simulink model "Ae483_project"  (R2018a)
settings: Solver=ode15s  StartTime=0.0  StopTime=50  RelTol=1e-4
values from neighbouring files (symbols this model uses):
  A_10_ang = [-1.3336 -0.5124 0.1399 ... (first row only)    [Ae483Project.m]
  A_10_ang_ob = bsxfun(@times, A_10_ang, [1.02; 1.04; 1.06])    [Ae483Project.m]
  A_10_full = [-0.006289	0.032720	1.318244	-32.063538	0.001827	-0.977238	0.000000	0.000733 ... (first row only)    [Ae483Project.m]
  A_80_ang = [-1.4979 -0.2372 0.4009 ... (first row only)    [Ae483Project.m]
  A_80_ang_ob = bsxfun(@times, A_80_ang, [1.02; 1.04; 1.06])    [Ae483Project.m]
  A_80_full = [-0.107611	0.120068	11.216902	-32.054340	0.007203	-0.521417	0.000000	-0.035677 ... (first row only)    [Ae483Project.m]
  B_10_ang = [-0.1712 16.8793 3.8113 ... (first row only)    [Ae483Project.m]
  B_10_ang_ob = bsxfun(@times, B_10_ang, [1.02; 1.04; 1.06])    [Ae483Project.m]
  B_10_full = [32.104822	29.961036	0.359934	0.000000 ... (first row only)    [Ae483Project.m]
  B_80_ang = [3.4190 17.0171 5.3246 ... (first row only)    [Ae483Project.m]
  B_80_ang_ob = bsxfun(@times, B_80_ang, [1.02; 1.04; 1.06])    [Ae483Project.m]
  B_80_full = [17.121858	64.081477	0.195110	0.000000 ... (first row only)    [Ae483Project.m]
  K_10 = B_10_ang^-1*(A_10_ang-A_d_ang)*C_ang^-1    [Ae483Project.m]
  K_80 = B_80_ang^-1*(A_80_ang-A_d_ang)*C_ang^-1    [Ae483Project.m]
  Ke_ang_10 = double(sym([ke1_ang_10; ke2_ang_10; ke3_ang_10]))    [Ae483Project.m]
  Ke_ang_80 = double(sym([ke1_ang_80; ke2_ang_80; ke3_ang_80]))    [Ae483Project.m]
  L_bv_10 = [cos(theta_10)*cos(psi_10), cos(theta_10)*sin(psi_10), -sin(theta_10) ... (first row only)    [Ae483Project.m]
  L_vb_10 = L_bv_10'    [Ae483Project.m]
undefined symbols (not defined in the file or in its folder): K_lqr_10, K_lqr_10_full, K_lqr_80, K_lqr_80_full
(part 1 of 2)
settings Model: Creator=90554  LastModifiedBy=90554

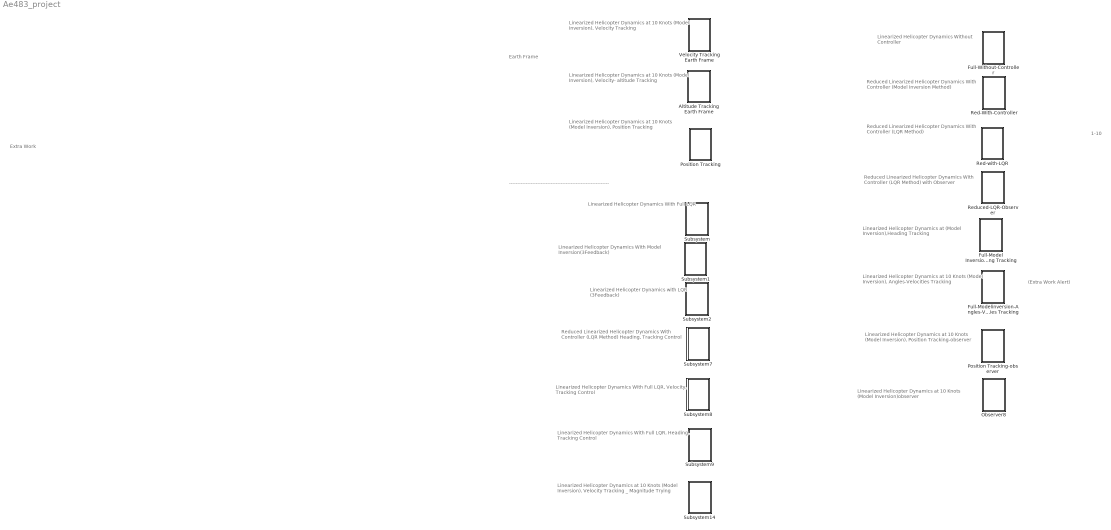
== system Ae483_project ==
  note: ------------------------------------------------------------
  note: (Extra Work Alert)
  note: 1-10
  note: Linearized Helicopter
      | Dynamics
      | Without Controller
  note: Reduced Linearized Helicopter
      | Dynamics
      | With Controller
      | (Model Inversion Method)
  note: Reduced Linearized Helicopter
      | Dynamics
      | With Controller
      | (LQR Method)
  note: Reduced Linearized Helicopter
      | Dynamics
      | With Controller
      | (LQR Method) with Observer
  note: Linearized Helicopter
      | Dynamics at
      | (Model Inversion),Heading Tracking
  note: Linearized Helicopter
      | Dynamics at 10 Knots
      | (Model Inversion), Angles-Velocities Tracking
  note: Linearized Helicopter
      | Dynamics at 10 Knots
      | (Model Inversion), Velocity Tracking
  note: Earth Frame
  note: Linearized Helicopter
      | Dynamics at 10 Knots
      | (Model Inversion), Velocity- altitude Tracking
  note: Reduced Linearized Helicopter
      | Dynamics
      | With Controller
      | (LQR Method) Heading, Tracking Control
  note: Linearized Helicopter
      | Dynamics
      | With Full LQR, Heading, Tracking Control
  note: Linearized Helicopter
      | Dynamics
      | With Full LQR, Velocity, Tracking Control
  note: Linearized Helicopter
      | Dynamics with
      | LQR (3Feedback)
  note: Linearized Helicopter
      | Dynamics
      | With Model Inversion(3Feedback)
  note: Linearized Helicopter
      | Dynamics
      | With Full LQR
  note: Linearized Helicopter
      | Dynamics at 10 Knots
      | (Model Inversion), Velocity Tracking _ Magnitude Trying
  note: Extra Work
  note: Linearized Helicopter
      | Dynamics at 10 Knots
      | (Model Inversion), Position Tracking
  note: Linearized Helicopter
      | Dynamics at 10 Knots
      | (Model Inversion), Position Tracking-observer
  note: Linearized Helicopter
      | Dynamics at 10 Knots
      | (Model Inversion)observer
  Altitude Tracking Earth Frame : Subsystem
  Full-Model Inversion-Heading Tracking : Subsystem
  Full-Modelinversion-Angles-Velocities Tracking : Subsystem
  Full-Without-Controller : Subsystem
  Observer8 : Subsystem
  Position Tracking : Subsystem
  Position Tracking-observer : Subsystem
  Red-With-Controller : Subsystem
  Red-with-LQR : Subsystem
  Reduced-LQR-Observer : Subsystem
  Subsystem : Subsystem
  Subsystem1 : Subsystem
  Subsystem14 : Subsystem
  Subsystem2 : Subsystem
  Subsystem7 : Subsystem
  Subsystem8 : Subsystem
  Subsystem9 : Subsystem
  Velocity Tracking Earth Frame : Subsystem

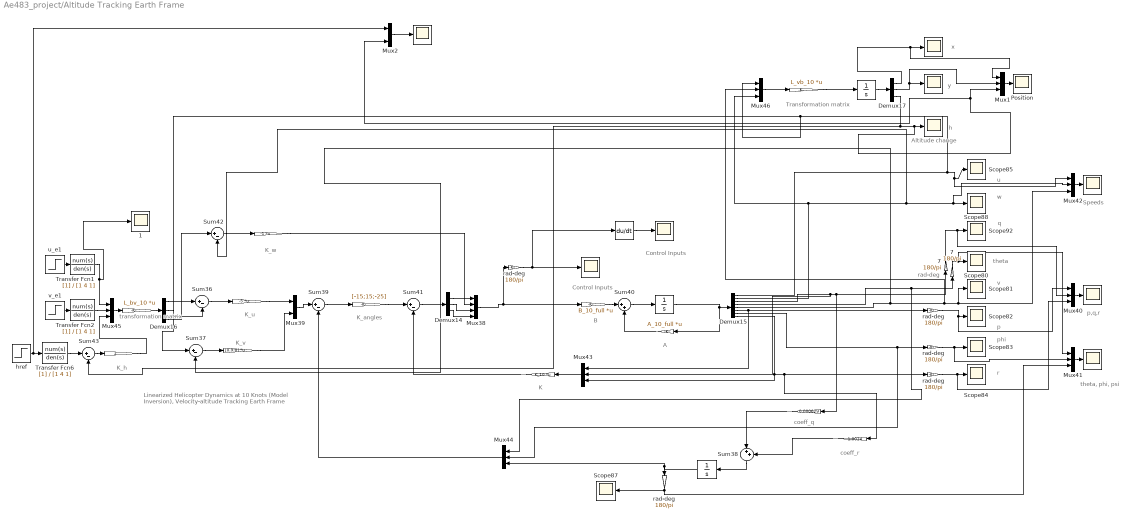
== system Ae483_project/Altitude Tracking Earth Frame ==
  note: x
  note: y
  note: h
  note: Transformation
      |       matrix
  note: Altitude change
  note: K_angles
  note: K_u
  note: K_w
  note: K_v
  note: transformation
      |      matrix
  note: K_h
  note: coeff_r
  note: coeff_q
  note: Control Inputs
  note: Control Inputs
  note: B
  note: K
  note: Linearized Helicopter
      | Dynamics at 10 Knots
      | (Model Inversion), Velocity-altitude Tracking Earth Frame
  note: w
  note: u
  note: p,q,r
  note: Speeds
  note: A
  note: phi
  note: theta
  note: p
  note: rad-deg
  note: theta, phi, psi
  note: r
  note: v
  note: q
  "    " : Gain  Gain=B_10_full  Multiplication=Matrix(K*u)
  "     " : Gain  Gain=2
  "       " : Gain  Gain=K_10  Multiplication=Matrix(K*u)
  "            " : Scope
  "             " : Integrator
  "              " : Scope
  "                " : Gain  Gain=1.0024
  "                    " : Gain  Gain=-1  Multiplication=Matrix(K*u)
  "                           " : Gain  Gain=A_10_full  Multiplication=Matrix(K*u)
  "                                    " : Gain  Gain=0.000629
  "                                      " : Gain  Gain=L_bv_10  Multiplication=Matrix(K*u)
  "                                              " : Integrator
  "                                               " : Derivative
  "                                                " : Scope
  "                                                          " : Scope
  "                                                                     " : Scope
  "                                                                        " : Integrator
  "                                                                         " : Gain  Gain=-5  Multiplication=Matrix(K*u)
  "                                                                                " : Gain  Gain=[-15;15;-25]
  "                                                                                 " : Scope
  "                                                                                   " : Scope
  "                                                                                     " : Scope
  "                                                                                       " : Scope
  "                                                                                        " : Gain  Gain=[0.9;0]  Multiplication=Matrix(K*u)
  "                                                                                                                                                      " : Gain  Gain=L_vb_10  Multiplication=Matrix(K*u)
  "                                                          1" : Scope
  "                                        Position                                            " : Scope
  "    7" : Gain  Gain=180/pi
  " 7" : Gain  Gain=180/pi
  " rad-deg   " : Gain  Gain=180/pi
  Demux14 : Demux  Outputs=3
  Demux15 : Demux  Outputs=8
  Demux16 : Demux  Outputs=3
  Demux17 : Demux  Outputs=3
  Mux{1,40..46} (8 alike) : Mux  Inputs=3
  Mux2 : Mux  Inputs=2
  Mux38 : Mux
  Mux39 : Mux  Inputs=2
  Scope{80..85,87..88,92} (9 alike) : Scope
  Sum{36..37,39,41..43} (6 alike) : Sum  Inputs=|+-
  Sum38 : Sum  Inputs=|++
  Sum40 : Sum  Inputs=|++
  Transfer Fcn1 : TransferFcn  Denominator=[1 4 1]
  Transfer Fcn2 : TransferFcn  Denominator=[1 4 1]
  Transfer Fcn6 : TransferFcn  Denominator=[1 4 1]
  href : Step  After=100  SampleTime=0
  "rad-deg  " : Gain  Gain=180/pi
  "rad-deg    " : Gain  Gain=180/pi
  "rad-deg     " : Gain  Gain=180/pi
  "rad-deg      " : Gain  Gain=180/pi
  u_e1 : Step  After=10  SampleTime=0
  v_e1 : Step  After=5  SampleTime=0
  wires:
  Demux14/2 -> Mux38/3
  "rad-deg     "/1 -> Mux41/2, Scope83/1
  Demux17/2 -> Mux1/2, "                                                          "/1
  Demux15/2 -> Sum42/2, Mux42/2, Scope88/1, Mux46/3
  "                                      "/1 -> Demux16/1
  Demux17/3 -> Sum43/2, "                                                                                   "/1, Mux2/2, Mux1/3
  "rad-deg      "/1 -> Mux40/1, Scope82/1
  Transfer Fcn1/1 -> "                                                          1"/1, Mux45/1
  Mux40/1 -> "                                                                     "/1
  "rad-deg  "/1 -> "            "/1, "                                               "/1
  Demux15/3 -> "                                    "/1, " 7"/1, Mux43/2
  Sum36/1 -> "                                                                         "/1
  href/1 -> Mux2/1, Transfer Fcn6/1
  Mux38/1 -> "    "/1, "rad-deg  "/1
  Mux45/1 -> "                                      "/1
  Demux15/7 -> Mux44/2, "rad-deg     "/1
  Demux15/6 -> "rad-deg      "/1, Mux43/1
  Demux15/5 -> Sum37/2, Mux46/2, Mux42/3, Scope81/1
  Transfer Fcn2/1 -> Mux45/2
  "                                                                                                                                                      "/1 -> "             "/1
  "                                                                                "/1 -> Sum41/1
  Demux15/1 -> Mux46/1, Sum36/2, Scope85/1, Mux42/1
  u_e1/1 -> Transfer Fcn1/1
  Sum43/1 -> "     "/1
  Mux41/1 -> "                                                "/1
  "rad-deg    "/1 -> Mux40/3, Scope84/1
  "     "/1 -> Mux45/3
  v_e1/1 -> Transfer Fcn2/1
  Transfer Fcn6/1 -> Sum43/1
  Mux46/1 -> "                                                                                                                                                      "/1
  "                                                                        "/1 -> Demux15/1, "                           "/1
  "                                              "/1 -> Mux44/3, " rad-deg   "/1
  Demux15/8 -> Mux43/3, "                "/1, "rad-deg    "/1
  " 7"/1 -> Mux40/2, Scope92/1
  Mux39/1 -> Sum39/1
  "                "/1 -> Sum38/2
  Sum39/1 -> "                                                                                "/1
  "             "/1 -> Demux17/1
  "                                    "/1 -> Sum38/1
  Demux15/4 -> "    7"/1, Mux44/1
  Sum40/1 -> "                                                                        "/1
  Demux16/1 -> Sum36/1
  Mux42/1 -> "                                                                                 "/1
  "       "/1 -> Sum41/2
  Demux14/1 -> Mux38/1
  " rad-deg   "/1 -> Mux41/3, Scope87/1
  Sum37/1 -> "                                                                                        "/1
  Sum41/1 -> Demux14/1
  "                           "/1 -> Sum40/2
  Mux44/1 -> Sum39/2
  "                                                                         "/1 -> Mux39/1
  Demux14/3 -> Mux38/4
  "                                                                                        "/1 -> Mux39/2
  "    7"/1 -> Mux41/1, Scope80/1
  "                    "/1 -> Mux38/2
  "    "/1 -> Sum40/1
  Demux17/1 -> Mux1/1, "                                                                                       "/1
  Sum38/1 -> "                                              "/1
  Mux43/1 -> "       "/1
  Demux16/3 -> Sum42/1
  Sum42/1 -> "                    "/1
  Demux16/2 -> Sum37/1
  "                                               "/1 -> "              "/1
  Mux1/1 -> "                                        Position                                            "/1
  Mux2/1 -> "                                                                                     "/1

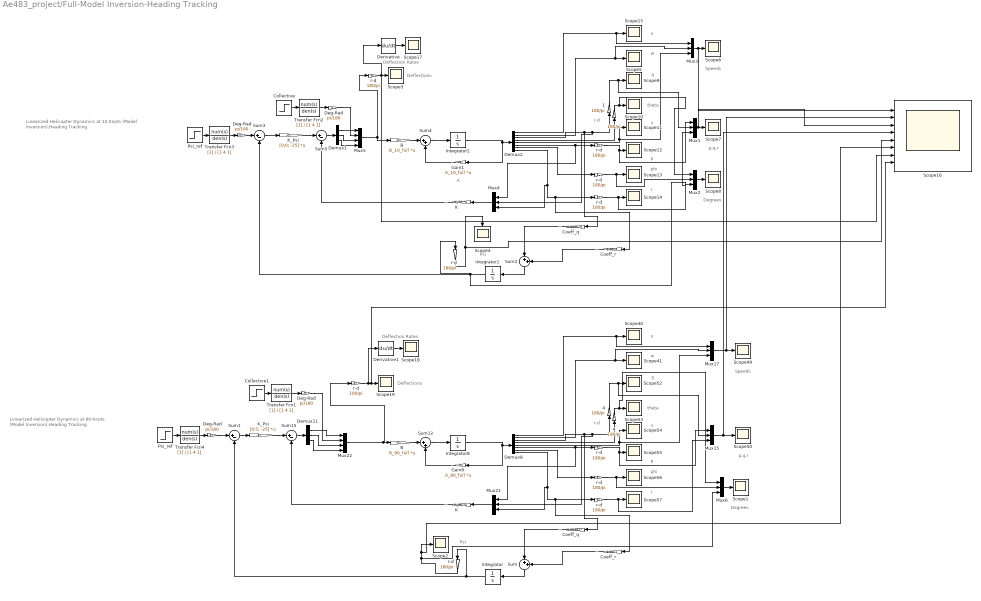
== system Ae483_project/Full-Model Inversion-Heading Tracking ==
  note: Deflection Rates
  note: Psi
  note: p,q,r
  note: A
  note: u
  note: phi
  note: Speeds
  note: r-d
  note: q
  note: r
  note: theta
  note: w
  note: p
  note: Linearized Helicopter
      | Dynamics at 80 Knots
      | (Model Inversion),Heading Tracking
  note: v
  note: v
  note: r
  note: p
  note: q
  note: Speeds
  note: Degrees
  note: phi
  note: r-d
  note: w
  note: A
  note: theta
  note: p,q,r
  note: Linearized Helicopter
      | Dynamics at 10 Knots
      | (Model Inversion),Heading Tracking
  note: u
  note: Deflections
  note: Deflections
  note: Deflection Rates
  note: Psi
  note: Degrees
  "      " : Gain  Gain=180/pi
  "           r-d              " : Gain  Gain=180/pi
  "        Coeff_q" : Gain  Gain=0.003617
  "        Coeff_r" : Gain  Gain=1.0027
  "    4" : Gain  Gain=180/pi
  "    Coeff_q" : Gain  Gain=0.000629
  "    Coeff_r" : Gain  Gain=1.0024
  "    K   " : Gain  Gain=K_10  Multiplication=Matrix(K*u)
  "    K     " : Gain  Gain=K_80  Multiplication=Matrix(K*u)
  "    K_Psi" : Gain  Gain=[0;0; -25]  Multiplication=Matrix(K*u)
  "    K_Psi " : Gain  Gain=[0;5; -25]  Multiplication=Matrix(K*u)
  "   r-d  " : Gain  Gain=180/pi
    Deg-Rad {,,,} (4 alike) : Gain  Gain=pi/180
  " 1" : Gain  Gain=180/pi
  " 4" : Gain  Gain=180/pi
  " r-d" : Gain  Gain=180/pi
  " r-d " : Gain  Gain=180/pi
  " r-d  " : Gain  Gain=180/pi
  " r-d   " : Gain  Gain=180/pi
  " r-d    " : Gain  Gain=180/pi
  " r-d     " : Gain  Gain=180/pi
  "B  " : Gain  Gain=B_10_full  Multiplication=Matrix(K*u)
  "B     " : Gain  Gain=B_80_full  Multiplication=Matrix(K*u)
  Collective : Step  After=5  SampleTime=0
  Collective1 : Step  After=5  SampleTime=0
  Demux1 : Demux  Outputs=3
  Demux11 : Demux  Outputs=3
  Demux2 : Demux  Outputs=8
  Demux8 : Demux  Outputs=8
  Derivative : Derivative
  Derivative1 : Derivative
  Gain1 : Gain  Gain=A_10_full  Multiplication=Matrix(K*u)
  Gain8 : Gain  Gain=A_80_full  Multiplication=Matrix(K*u)
  Integrator{,1..2,8} (4 alike) : Integrator
  Mux{1..4,6,15,17,21} (8 alike) : Mux  Inputs=3
  Mux22 : Mux
  Mux5 : Mux
  Psi_ref : Step  After=15  SampleTime=0
  "Psi_ref  " : Step  After=15  SampleTime=0
  Scope{1..15,17..19,40..41,49..50,52..57} (28 alike) : Scope
  Scope16 : Scope  NumInputPorts=8
  Sum{,2,4,12} (4 alike) : Sum  Inputs=|++
  Sum{1,3,5,15} (4 alike) : Sum  Inputs=|+-
  Transfer Fcn{1..4} (4 alike) : TransferFcn  Denominator=[1 4 1]
  "r-d " : Gain  Gain=180/pi
  "r-d    " : Gain  Gain=180/pi
  wires:
  Mux5/1 -> "B  "/1, " r-d    "/1
  "    Coeff_r"/1 -> Sum2/2
  "    K_Psi "/1 -> Sum15/1
  " 1"/1 -> Mux1/2, Scope9/1
  Integrator/1 -> Sum1/2, " r-d "/1
  Demux8/8 -> Mux21/3, "        Coeff_r"/1, "   r-d  "/1
  "        Coeff_r"/1 -> Sum/2
  " r-d "/1 -> Mux6/3, Scope16/6, Scope2/1
  " r-d   "/1 -> Mux2/2, Scope13/1
  Transfer Fcn3/1 -> "  Deg-Rad "/1
  Mux22/1 -> "B     "/1, "           r-d              "/1
  Demux2/8 -> Mux4/3, "    Coeff_r"/1, " r-d     "/1
  " r-d  "/1 -> Mux6/2, Scope56/1
  Demux8/3 -> "        Coeff_q"/1, Mux21/2, " 4"/1
  "r-d "/1 -> Mux15/1, Scope55/1
  Mux17/1 -> Scope16/2, Scope49/1
  Demux11/1 -> Mux22/1
  Demux8/5 -> Mux17/3, Scope54/1
  Demux1/1 -> Mux5/1
  Demux1/3 -> Mux5/4
  Sum3/1 -> "    K_Psi"/1
  Demux8/6 -> Mux21/1, "r-d "/1
  " 4"/1 -> Mux15/2, Scope52/1
  Mux1/1 -> Scope16/3, Scope7/1
  Sum5/1 -> Demux1/1
  Sum12/1 -> Integrator8/1
  Demux8/1 -> Mux17/1, Scope40/1
  " r-d     "/1 -> Mux1/3, Scope14/1
  "    4"/1 -> Mux6/1, Scope53/1
  "  Deg-Rad "/1 -> Mux5/2
  Sum4/1 -> Integrator2/1
  Mux15/1 -> Scope16/4, Scope50/1
  "B  "/1 -> Sum4/1
  Collective/1 -> Transfer Fcn2/1
  Demux2/5 -> Mux3/3, Scope11/1
  Demux11/3 -> Mux22/4
  "   r-d  "/1 -> Mux15/3, Scope57/1
  Gain8/1 -> Sum12/2
  Integrator1/1 -> " r-d"/1, Mux2/3, Sum3/2
  "    K   "/1 -> Sum5/2
  Sum/1 -> Integrator/1
  Demux2/1 -> Scope15/1, Mux3/1
  Demux1/2 -> Mux5/3
  " r-d    "/1 -> Scope16/7, Derivative/1, Scope3/1
  Sum1/1 -> "    K_Psi "/1
  Mux3/1 -> Scope16/1, Scope6/1
  Demux2/2 -> Mux3/2, Scope5/1
  Demux8/4 -> "    4"/1
  Gain1/1 -> Sum4/2
  "        Coeff_q"/1 -> Sum/1
  "    K     "/1 -> Sum15/2
  "    K_Psi"/1 -> Sum5/1
  Demux2/7 -> " r-d   "/1
  Demux2/4 -> "      "/1
  " r-d"/1 -> Scope16/5, Scope4/1
  "B     "/1 -> Sum12/1
  Integrator2/1 -> Demux2/1, Gain1/1
  Demux2/6 -> Mux4/1, "r-d    "/1
  "r-d    "/1 -> Mux1/1, Scope12/1
  Sum2/1 -> Integrator1/1
  Mux4/1 -> "    K   "/1
  Demux8/2 -> Mux17/2, Scope41/1
  Demux8/7 -> " r-d  "/1
  Demux2/3 -> "    Coeff_q"/1, Mux4/2, " 1"/1
  Demux11/2 -> Mux22/3
  "           r-d              "/1 -> Derivative1/1, Scope16/8, Scope19/1
  Integrator8/1 -> Demux8/1, Gain8/1
  Psi_ref/1 -> Transfer Fcn3/1
  "  Deg-Rad "/1 -> Sum3/1
  "      "/1 -> Mux2/1, Scope10/1
  Mux2/1 -> Scope8/1
  Mux21/1 -> "    K     "/1
  Sum15/1 -> Demux11/1
  "    Coeff_q"/1 -> Sum2/1
  Transfer Fcn2/1 -> "  Deg-Rad "/1
  Derivative/1 -> Scope17/1
  Derivative1/1 -> Scope18/1
  Collective1/1 -> Transfer Fcn1/1
  Transfer Fcn1/1 -> "  Deg-Rad "/1
  "  Deg-Rad "/1 -> Mux22/2
  Transfer Fcn4/1 -> "  Deg-Rad "/1
  "Psi_ref  "/1 -> Transfer Fcn4/1
  "  Deg-Rad "/1 -> Sum1/1
  Mux6/1 -> Scope1/1

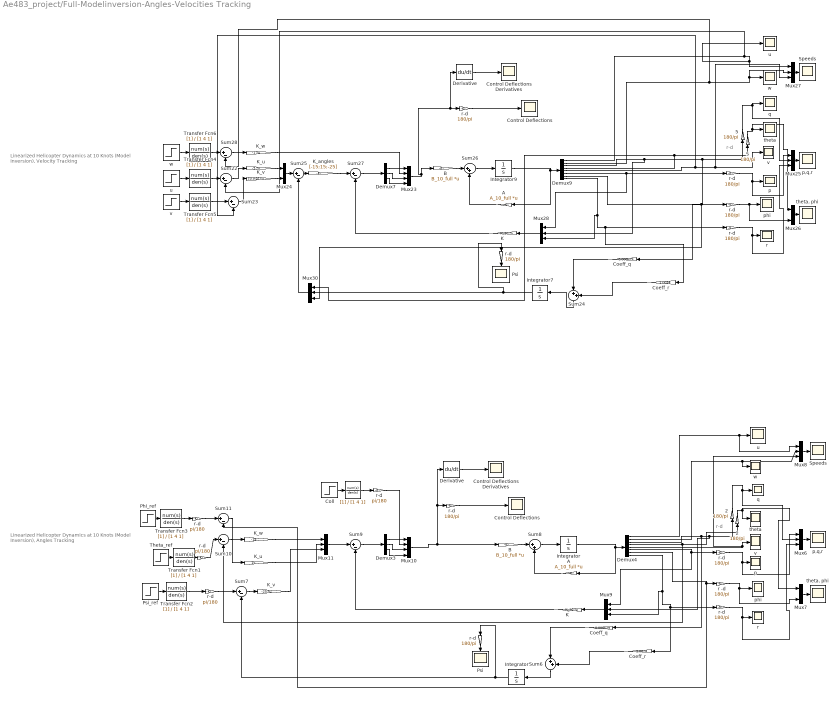
== system Ae483_project/Full-Modelinversion-Angles-Velocities Tracking ==
  note: r-d
  note: Linearized Helicopter
      | Dynamics at 10 Knots
      | (Model Inversion), Angles Tracking
  note: r-d
  note: Linearized Helicopter
      | Dynamics at 10 Knots
      | (Model Inversion), Velocity Tracking
  "  " : TransferFcn  Denominator=[1 4 1]
  "                K   " : Gain  Gain=K_10  Multiplication=Matrix(K*u)
  "        A   " : Gain  Gain=A_10_full  Multiplication=Matrix(K*u)
  "      K " : Gain  Gain=K_10  Multiplication=Matrix(K*u)
  "      K_u  " : Gain  Gain=15
  "      K_v  " : Gain  Gain=-25  Multiplication=Matrix(K*u)
  "      r-d   " : Gain  Gain=180/pi
  "      r-d        " : Gain  Gain=pi/180
  "     K_w  " : Gain  Gain=-15
  "    2" : Gain  Gain=180/pi
  "    5" : Gain  Gain=180/pi
  "    Coeff_q" : Gain  Gain=0.000629
  "    Coeff_q  " : Gain  Gain=0.000629
  "    Coeff_r" : Gain  Gain=1.0024
  "    Coeff_r   " : Gain  Gain=1.0024
  "    K_angles" : Gain  Gain=[-15;15;-25]
  "    K_u" : Gain  Gain=-5  Multiplication=Matrix(K*u)
  "    K_v" : Gain  Gain=[0.9;0]  Multiplication=Matrix(K*u)
  "    K_w" : Gain  Gain=-1  Multiplication=Matrix(K*u)
  "    r-d   " : Gain  Gain=180/pi
  "    r-d     " : Gain  Gain=180/pi
  "   r-d   " : Gain  Gain=pi/180
  "   r-d    " : Gain  Gain=180/pi
  "   r-d     " : Gain  Gain=180/pi
  "   r-d      " : Gain  Gain=pi/180
  "  B  " : Gain  Gain=B_10_full  Multiplication=Matrix(K*u)
  "  Control Deflections  " : Scope
  "  Control Deflections Derivatives" : Scope
  "  Control Deflections Derivatives  " : Scope
  "  Control Deflections    " : Scope
  "  Derivative" : Derivative
  "  Derivative  " : Derivative
  "  Integrator" : Integrator
  "  p" : Scope
  "  p,q,r  " : Scope
  "  phi  " : Scope
  "  r-d   " : Gain  Gain=180/pi
  "  r-d    " : Gain  Gain=180/pi
  "  theta" : Scope
  "  u" : Scope
  "  v" : Scope
  "  w" : Scope
  " 2" : Gain  Gain=180/pi
  " 5" : Gain  Gain=180/pi
  " Speeds  " : Scope
  " q  " : Scope
  " r  " : Scope
  " r -d" : Gain  Gain=180/pi
  " r-d  " : Gain  Gain=pi/180
  " r-d    " : Gain  Gain=180/pi
  " theta, phi  " : Scope
  A : Gain  Gain=A_10_full  Multiplication=Matrix(K*u)
  B : Gain  Gain=B_10_full  Multiplication=Matrix(K*u)
  "Coll    " : Step  After=5  SampleTime=0
  Demux3 : Demux  Outputs=3
  Demux4 : Demux  Outputs=8
  Demux7 : Demux  Outputs=3
  Demux9 : Demux  Outputs=8
  Integrator : Integrator
  Integrator7 : Integrator
  Integrator9 : Integrator
  Mux10 : Mux
  Mux{6,8..9,11,25,27..28,30} (8 alike) : Mux  Inputs=3
  Mux23 : Mux
  Mux24 : Mux  Inputs=2
  Mux26 : Mux  Inputs=2
  Mux7 : Mux  Inputs=2
  Phi_ref : Step  After=8  SampleTime=0
  Psi : Scope
  "Psi " : Scope
  Psi_ref : Step  After=15  SampleTime=0
  Speeds : Scope
  Sum{7,9..11,22..23,25,27..28} (9 alike) : Sum  Inputs=|+-
  Sum{6,8,24,26} (4 alike) : Sum  Inputs=|++
  Theta_ref : Step  After=5  SampleTime=0
  Transfer Fcn{1..6} (6 alike) : TransferFcn  Denominator=[1 4 1]
  p : Scope
  p,q,r : Scope
  phi : Scope
  q : Scope
  r : Scope
  "r-d     " : Gain  Gain=180/pi
  theta : Scope
  "theta, phi" : Scope
  u : Scope
  "u " : Step  After=5  SampleTime=0
  v : Scope
  "v  " : Step  After=15  SampleTime=0
  w : Scope
  "w  " : Step  After=8  SampleTime=0
  wires:
  "   r-d   "/1 -> Sum7/1
  Sum28/1 -> "    K_w"/1
  Demux4/6 -> Mux9/1, "r-d     "/1
  "    Coeff_q"/1 -> Sum24/1
  Mux11/1 -> Sum9/1
  Demux7/3 -> Mux23/4
  "   r-d     "/1 -> Mux25/3, r/1
  "    Coeff_r"/1 -> Sum24/2
  "      r-d   "/1 -> "Psi "/1
  Sum10/1 -> "     K_w  "/1
  Sum8/1 -> Integrator/1
  Demux4/5 -> Mux8/3, "  v"/1
  Integrator7/1 -> " r-d    "/1, Mux30/3
  "    K_w"/1 -> Mux23/2
  "  Integrator"/1 -> Sum7/2, "      r-d   "/1
  Integrator9/1 -> Demux9/1, A/1
  Demux9/4 -> "    5"/1, Mux30/1
  Demux4/1 -> "  u"/1, Mux8/1
  "  r-d    "/1 -> Mux6/3, " r  "/1
  Integrator/1 -> Demux4/1, "        A   "/1
  " r -d"/1 -> Mux7/2, "  phi  "/1
  Demux4/4 -> "    2"/1, Sum10/2
  "     K_w  "/1 -> Mux11/1
  "    K_u"/1 -> Mux24/1
  " r-d    "/1 -> Psi/1
  Demux4/3 -> "    Coeff_q  "/1, Mux9/2, " 2"/1
  Demux7/1 -> Mux23/1
  Sum27/1 -> Demux7/1
  "      K_v  "/1 -> Mux11/3
  Mux27/1 -> Speeds/1
  Mux9/1 -> "                K   "/1
  B/1 -> Sum26/1
  Mux6/1 -> "  p,q,r  "/1
  Demux4/2 -> Mux8/2, "  w"/1
  "   r-d    "/1 -> Mux26/2, phi/1
  " 2"/1 -> Mux6/2, " q  "/1
  Sum23/1 -> "    K_v"/1
  "Coll    "/1 -> "  "/1
  Demux4/7 -> " r -d"/1, Sum11/2
  "        A   "/1 -> Sum8/2
  "r-d     "/1 -> Mux6/1, "  p"/1
  "    Coeff_r   "/1 -> Sum6/2
  "      K_u  "/1 -> Mux11/2
  "    Coeff_q  "/1 -> Sum6/1
  Demux9/7 -> Mux30/2, "   r-d    "/1
  "   r-d      "/1 -> Mux10/2
  Demux4/8 -> Mux9/3, "    Coeff_r   "/1, "  r-d    "/1
  "      r-d        "/1 -> Sum11/1
  Demux3/2 -> Mux10/3
  Demux3/1 -> Mux10/1
  Demux7/2 -> Mux23/3
  Sum7/1 -> "      K_v  "/1
  Sum6/1 -> "  Integrator"/1
  Demux9/5 -> Sum23/2, v/1, Mux27/3
  "  B  "/1 -> Sum8/1
  " 5"/1 -> Mux25/2, q/1
  Sum9/1 -> Demux3/1
  Demux3/3 -> Mux10/4
  "  "/1 -> "   r-d      "/1
  " r-d  "/1 -> Sum10/1
  Demux9/3 -> "    Coeff_q"/1, " 5"/1, Mux28/2
  "    5"/1 -> Mux26/1, theta/1
  Mux26/1 -> "theta, phi"/1
  Sum24/1 -> Integrator7/1
  Demux9/2 -> Sum28/2, Mux27/2, w/1
  "    r-d     "/1 -> Mux25/1, p/1
  Demux9/6 -> Mux28/1, "    r-d     "/1
  Demux9/1 -> Sum22/2, u/1, Mux27/1
  Sum11/1 -> "      K_u  "/1
  Mux7/1 -> " theta, phi  "/1
  Sum26/1 -> Integrator9/1
  Demux9/8 -> Mux28/3, "    Coeff_r"/1, "   r-d     "/1
  "    K_angles"/1 -> Sum27/1
  Mux25/1 -> p,q,r/1
  "      K "/1 -> Sum27/2
  "    2"/1 -> Mux7/1, "  theta"/1
  Mux30/1 -> Sum25/2
  Mux24/1 -> Sum25/1
  "                K   "/1 -> Sum9/2
  Mux28/1 -> "      K "/1
  Mux8/1 -> " Speeds  "/1
  "    K_v"/1 -> Mux24/2
  Sum25/1 -> "    K_angles"/1
  Sum22/1 -> "    K_u"/1
  A/1 -> Sum26/2
  "  Derivative"/1 -> "  Control Deflections Derivatives"/1
  Mux23/1 -> B/1, "  Derivative"/1, "  r-d   "/1
  "  r-d   "/1 -> "  Control Deflections  "/1
  "  Derivative  "/1 -> "  Control Deflections Derivatives  "/1
  Mux10/1 -> "  Derivative  "/1, "    r-d   "/1, "  B  "/1
  "    r-d   "/1 -> "  Control Deflections    "/1
  Transfer Fcn3/1 -> "      r-d        "/1
  Transfer Fcn1/1 -> " r-d  "/1
  Transfer Fcn2/1 -> "   r-d   "/1
  Phi_ref/1 -> Transfer Fcn3/1
  Theta_ref/1 -> Transfer Fcn1/1
  Psi_ref/1 -> Transfer Fcn2/1
  "u "/1 -> Transfer Fcn4/1
  Transfer Fcn4/1 -> Sum22/1
  Transfer Fcn5/1 -> Sum23/1
  "v  "/1 -> Transfer Fcn5/1
  "w  "/1 -> Transfer Fcn6/1
  Transfer Fcn6/1 -> Sum28/1

== system Ae483_project/Full-Without-Controller ==
  note: Linearized Helicopter
      | Dynamics at 10 Knots
      | Without Controller
  note: A
  note: R-D
  note: Linearized Helicopter
      | Dynamics at 80 Knots
      | Without Controller
  note: A
  note: r-d
  " " : Gain  Gain=180/pi
  "    " : Gain  Gain=180/pi
  "               " : Gain  Gain=180/pi
  " 1" : Gain  Gain=180/pi
  " R-D" : Gain  Gain=180/pi
  " R-D   " : Gain  Gain=180/pi
  " r-d   " : Gain  Gain=180/pi
  " r-d         " : Gain  Gain=180/pi
  " u    " : Scope
  B : Gain  Gain=B_10_full  Multiplication=Matrix(K*u)
  "B   " : Gain  Gain=B_80_full  Multiplication=Matrix(K*u)
  Collective : Step  After=10  SampleTime=0
  "Collective  " : Step  After=10  SampleTime=0
  Deg-Rad : Gain  Gain=pi/180
  "Deg-Rad   " : Gain  Gain=pi/180
  Demux : Demux  Outputs=8
  Demux1 : Demux  Outputs=8
  Gain : Gain  Gain=A_10_full  Multiplication=Matrix(K*u)
  Gain1 : Gain  Gain=A_80_full  Multiplication=Matrix(K*u)
  Integrator : Integrator
  Integrator1 : Integrator
  Lat_Cyc : Step  After=0  SampleTime=0
  "Lat_Cyc  " : Step  After=0  SampleTime=0
  Long_Cyc : Step  After=0  SampleTime=0
  "Long_Cyc  " : Step  After=0  SampleTime=0
  Mux : Mux
  Mux1 : Mux
  Mux33 : Mux  Inputs=2
  Mux{6,8,34..35} (4 alike) : Mux  Inputs=3
  Mux7 : Mux  Inputs=2
  Pedal : Step  After=0  SampleTime=0
  "Pedal  " : Step  After=0  SampleTime=0
  Phi : Scope
  "R-D    " : Gain  Gain=180/pi
  Speeds : Scope
  "Speeds   " : Scope
  Sum : Sum  Inputs=|++
  Sum1 : Sum  Inputs=|++
  "Theta " : Scope
  Theta Phi : Scope
  V : Scope
  p : Scope
  "p   " : Scope
  p q r : Scope
  "p,q,r " : Scope
  phi : Scope
  q : Scope
  "q  " : Scope
  r : Scope
  "r  " : Scope
  "r-d     " : Gain  Gain=180/pi
  theta : Scope
  "theta, phi" : Scope
  "u " : Scope
  "v " : Scope
  w : Scope
  "w  " : Scope
  wires:
  Integrator/1 -> Demux/1, Gain/1
  Mux1/1 -> "Deg-Rad   "/1
  " 1"/1 -> Mux34/2, "q  "/1
  Demux1/5 -> Mux35/3, "v "/1
  Demux/5 -> Mux8/3, V/1
  Mux34/1 -> "p,q,r "/1
  Lat_Cyc/1 -> Mux/3
  Demux1/4 -> "               "/1
  "Deg-Rad   "/1 -> "B   "/1
  " r-d   "/1 -> Mux34/3, "r  "/1
  " "/1 -> Mux6/2, q/1
  Collective/1 -> Mux/2
  Long_Cyc/1 -> Mux/1
  Demux/4 -> "    "/1
  "               "/1 -> Mux33/1, "Theta "/1
  Sum1/1 -> Integrator1/1
  " R-D   "/1 -> r/1, Mux6/3
  Demux/1 -> Mux8/1, " u    "/1
  "R-D    "/1 -> Mux6/1, p/1
  " R-D"/1 -> Mux7/2, Phi/1
  Demux1/8 -> " r-d   "/1
  Demux/6 -> "R-D    "/1
  Demux1/6 -> "r-d     "/1
  Pedal/1 -> Mux/4
  Sum/1 -> Integrator/1
  "r-d     "/1 -> Mux34/1, "p   "/1
  Mux33/1 -> "theta, phi"/1
  Gain1/1 -> Sum1/2
  Deg-Rad/1 -> B/1
  Mux/1 -> Deg-Rad/1
  Gain/1 -> Sum/2
  Integrator1/1 -> Demux1/1, Gain1/1
  " r-d         "/1 -> Mux33/2, phi/1
  Demux1/7 -> " r-d         "/1
  Demux/7 -> " R-D"/1
  Demux1/3 -> " 1"/1
  B/1 -> Sum/1
  Mux7/1 -> Theta Phi/1
  Demux1/2 -> Mux35/2, "w  "/1
  Demux/8 -> " R-D   "/1
  "B   "/1 -> Sum1/1
  Demux1/1 -> Mux35/1, "u "/1
  Mux8/1 -> Speeds/1
  Demux/2 -> Mux8/2, w/1
  Mux6/1 -> p q r/1
  Mux35/1 -> "Speeds   "/1
  "    "/1 -> Mux7/1, theta/1
  Demux/3 -> " "/1
  "Lat_Cyc  "/1 -> Mux1/3
  "Collective  "/1 -> Mux1/2
  "Pedal  "/1 -> Mux1/4
  "Long_Cyc  "/1 -> Mux1/1

== system Ae483_project/Observer8 ==
  note: r-d
  note: phi
  note: p
  note: r
  note: q
  note: v
  note: Collective
  note: Speeds
  note: Long_Cyc
  note: Pedal
  note: w
  note: theta
  note: u
  note: p,q,r
  note: A
  note: Lat_Cyc
  note: y_ob
  note: x_dot_ob
  note: x_ob
  note: theta, phi
  "       " : Gain  Gain=180/pi
  "    K   " : Gain  Gain=K_10  Multiplication=Matrix(K*u)
  " 8" : Gain  Gain=180/pi
  " r-d  " : Gain  Gain=180/pi
  " r-d     " : Gain  Gain=180/pi
  "A_ob      " : Gain  Gain=A_10_ang_ob  Multiplication=Matrix(K*u)
  "B  " : Gain  Gain=B_10_full  Multiplication=Matrix(K*u)
  "B_ob     " : Gain  Gain=B_10_ang_ob  Multiplication=Matrix(K*u)
  Demux15 : Demux  Outputs=3
  Demux16 : Demux  Outputs=8
  Demux17 : Demux  Outputs=3
  "Error p, in degree1" : Scope
  Gain2 : Gain  Gain=A_10_full  Multiplication=Matrix(K*u)
  Integrator3 : Integrator
  Integrator4 : Integrator
  "Ke      " : Gain  Description=K  Gain=Ke_ang_10  Multiplication=Matrix(K*u)
  Mux{42,44..46} (4 alike) : Mux  Inputs=3
  Mux43 : Mux  Inputs=2
  Mux47 : Mux
  "Rad-Deg  " : Gain  Gain=pi/180
  Scope{1..3,9..11,15,17..19,64..65} (12 alike) : Scope
  Step{1..4} (4 alike) : Step  After=5  SampleTime=0
  Sum18 : Sum  Inputs=|++-
  Sum2 : Sum  Inputs=|++
  Sum8 : Sum  Inputs=|+-
  Sum9 : Sum  Inputs=|+-
  Transfer Fcn{20..23} (4 alike) : TransferFcn  Denominator=[1 4 1]
  deg-r : Gain  Gain=pi/180
  "r-d      " : Gain  Gain=1800000/pi
  "r-d       " : Gain  Gain=180/pi
  wires:
  Mux47/1 -> Scope9/1, "Rad-Deg  "/1
  Demux16/4 -> "       "/1
  Mux42/1 -> Scope2/1
  Mux46/1 -> "    K   "/1
  "       "/1 -> Mux43/1, Scope17/1
  Gain2/1 -> Sum2/2
  "r-d       "/1 -> Mux42/1, Scope19/1
  "B  "/1 -> Sum2/1
  Step2/1 -> Transfer Fcn23/1
  Demux16/6 -> Sum9/2, "r-d       "/1
  Step3/1 -> Transfer Fcn20/1
  Demux16/8 -> " r-d     "/1
  Demux15/3 -> Mux47/4
  Demux16/3 -> " 8"/1
  Demux15/2 -> Mux47/3
  Transfer Fcn23/1 -> Mux45/3
  Integrator3/1 -> Demux16/1, Gain2/1
  Demux16/7 -> " r-d  "/1
  "    K   "/1 -> Sum8/2
  Transfer Fcn22/1 -> Mux45/2
  Demux16/2 -> Mux44/2, Scope11/1
  Demux15/1 -> Mux47/1
  Demux16/5 -> Mux44/3, Scope18/1
  Mux43/1 -> Scope3/1
  " 8"/1 -> Mux42/2, Scope15/1
  Transfer Fcn20/1 -> Mux45/1
  Step1/1 -> Transfer Fcn22/1
  "Rad-Deg  "/1 -> "B  "/1
  " r-d     "/1 -> Mux42/3, Scope65/1
  Transfer Fcn21/1 -> Mux47/2
  Step4/1 -> Transfer Fcn21/1
  Demux17/2 -> Mux46/2
  deg-r/1 -> "B_ob     "/1
  "r-d      "/1 -> "Error p, in degree1"/1
  Sum18/1 -> Integrator4/1
  Mux45/1 -> Sum8/1
  Sum2/1 -> Integrator3/1
  Integrator4/1 -> Demux17/1, "A_ob      "/1
  Demux17/1 -> Mux46/1, Sum9/1
  "A_ob      "/1 -> Sum18/1
  Mux44/1 -> Scope1/1
  "B_ob     "/1 -> Sum18/2
  Sum9/1 -> "r-d      "/1, "Ke      "/1  "Error_y"
  " r-d  "/1 -> Mux43/2, Scope64/1
  Demux17/3 -> Mux46/3
  Demux16/1 -> Mux44/1, Scope10/1
  Sum8/1 -> deg-r/1, Demux15/1
  "Ke      "/1 -> Sum18/3

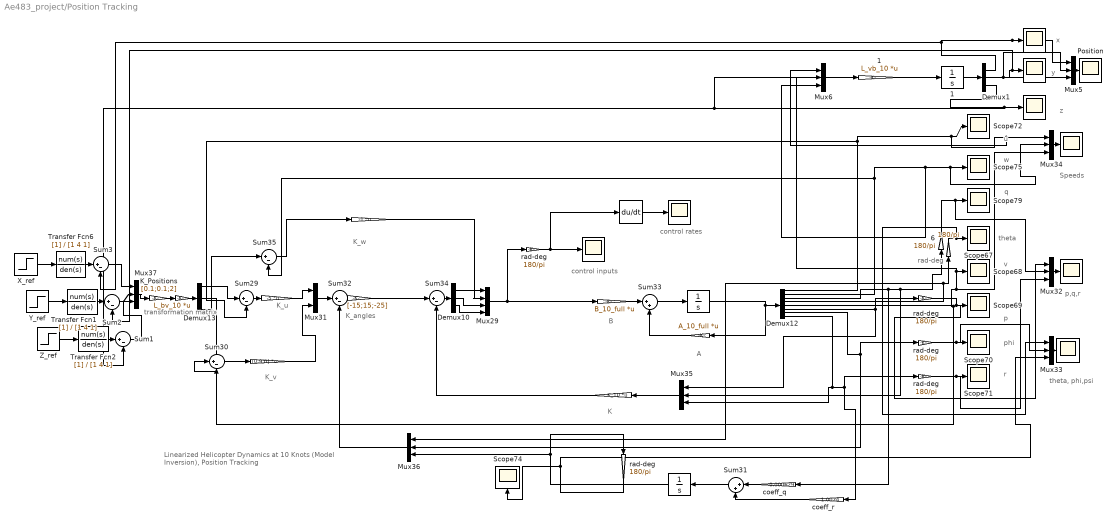
== system Ae483_project/Position Tracking ==
  note: z
  note: u
  note: q
  note: control rates
  note: K
  note: theta
  note: p
  note: B
  note: A
  note: K_w
  note: phi
  note: Speeds
  note: v
  note: w
  note: rad-deg
  note: r
  note: theta, phi,psi
  note: p,q,r
  note: control inputs
  note: K_angles
  note: K_u
  note: K_v
  note: transformation
      |        matrix
  note: Linearized Helicopter
      | Dynamics at 10 Knots
      | (Model Inversion), Position Tracking
  note: y
  note: x
  " " : Scope
  "   " : Integrator
  "    " : Gain  Gain=B_10_full  Multiplication=Matrix(K*u)
  "     " : Gain  Gain=180/pi
  "          " : Gain  Gain=A_10_full  Multiplication=Matrix(K*u)
  "                      " : Gain  Gain=K_10  Multiplication=Matrix(K*u)
  "                       " : Gain  Gain=[-15;15;-25]
  "                           " : Gain  Gain=L_bv_10  Multiplication=Matrix(K*u)
  "                                   " : Gain  Gain=-5  Multiplication=Matrix(K*u)
  "                                    " : Gain  Gain=[0.9;0]  Multiplication=Matrix(K*u)
  "                                     " : Derivative
  "                                         " : Scope
  "                                               " : Scope
  "                                                         " : Scope
  "                                                           " : Gain  Gain=-1  Multiplication=Matrix(K*u)
  "                                                               " : Scope
  "                                                                     " : Scope
  "                                                                                 " : Scope
  "                                                                                                       " : Scope
  "                                                                                                           " : Integrator
  "                                                                                                                                                      1" : Gain  Gain=L_vb_10  Multiplication=Matrix(K*u)
  "             1" : Integrator
  "    coeff_q" : Gain  Gain=0.000629
  "    coeff_r" : Gain  Gain=1.0024
  " 6" : Gain  Gain=180/pi
  " rad-deg       " : Gain  Gain=180/pi
  Demux1 : Demux  Outputs=3
  Demux10 : Demux  Outputs=3
  Demux12 : Demux  Outputs=8
  Demux13 : Demux  Outputs=3
  K_Positions : Gain  Gain=[0.1;0.1;2]
  Mux29 : Mux
  Mux31 : Mux  Inputs=2
  Mux{5..6,32..37} (8 alike) : Mux  Inputs=3
  Position : Scope
  Scope{67..72,74..75,79} (9 alike) : Scope
  Sum{1..3,29..30,32,34..35} (8 alike) : Sum  Inputs=|+-
  Sum31 : Sum  Inputs=|++
  Sum33 : Sum  Inputs=|++
  Transfer Fcn1 : TransferFcn  Denominator=[1 4 1]
  Transfer Fcn2 : TransferFcn  Denominator=[1 4 1]
  Transfer Fcn6 : TransferFcn  Denominator=[1 4 1]
  X_ref : Step  After=50  SampleTime=0
  Y_ref : Step  After=100  SampleTime=0
  Z_ref : Step  After=150  SampleTime=0
  rad-deg : Gain  Gain=180/pi
  "rad-deg  " : Gain  Gain=180/pi
  "rad-deg     " : Gain  Gain=180/pi
  "rad-deg        " : Gain  Gain=180/pi
  wires:
  "    coeff_r"/1 -> Sum31/2
  Sum35/1 -> "                                                           "/1
  Mux37/1 -> K_Positions/1
  Demux13/3 -> Sum35/1
  "rad-deg        "/1 -> Scope74/1, Mux33/3
  Demux12/6 -> Mux35/1, "rad-deg  "/1
  " rad-deg       "/1 -> Mux32/3, Scope71/1
  Demux1/3 -> Sum1/2, Mux5/3, "                                                               "/1
  Y_ref/1 -> Transfer Fcn1/1
  Mux33/1 -> "                                               "/1
  Demux12/4 -> "     "/1, Mux36/1
  Demux13/2 -> Sum30/1
  "rad-deg     "/1 -> " "/1, "                                     "/1
  Mux31/1 -> Sum32/1
  Demux12/1 -> Scope72/1, Mux6/1, Mux34/1, Sum29/2
  Transfer Fcn2/1 -> Sum1/1
  Demux12/8 -> Mux35/3, "    coeff_r"/1, " rad-deg       "/1
  "          "/1 -> Sum33/2
  "                           "/1 -> Demux13/1
  "    "/1 -> Sum33/1
  Sum32/1 -> "                       "/1
  Mux32/1 -> "                                                         "/1
  rad-deg/1 -> Mux33/2, Scope70/1
  Demux12/3 -> "    coeff_q"/1, Mux35/2, " 6"/1
  Mux35/1 -> "                      "/1
  "rad-deg  "/1 -> Mux32/1, Scope69/1
  Sum31/1 -> "                                                                                                           "/1
  "                                     "/1 -> "                                         "/1
  "                                                                                                           "/1 -> "rad-deg        "/1, Mux36/3
  "   "/1 -> Demux12/1, "          "/1
  " 6"/1 -> Mux32/2, Scope79/1
  "                                                                                                                                                      1"/1 -> "             1"/1
  K_Positions/1 -> "                           "/1
  X_ref/1 -> Transfer Fcn6/1
  Sum29/1 -> "                                   "/1
  "                                   "/1 -> Mux31/1
  Sum2/1 -> Mux37/2
  Demux1/2 -> Mux5/2, Sum2/2, "                                                                                 "/1
  "                                    "/1 -> Mux31/2
  Sum1/1 -> Mux37/3
  Sum30/1 -> "                                    "/1
  "     "/1 -> Mux33/1, Scope67/1
  Demux10/1 -> Mux29/1
  Mux6/1 -> "                                                                                                                                                      1"/1
  Demux10/3 -> Mux29/4
  Mux36/1 -> Sum32/2
  Demux12/7 -> rad-deg/1, Mux36/2
  Mux34/1 -> "                                                                     "/1
  "                      "/1 -> Sum34/2
  "                       "/1 -> Sum34/1
  Demux12/2 -> Mux6/3, Mux34/2, Scope75/1, Sum35/2
  Demux12/5 -> Mux34/3, Mux6/2, Scope68/1, Sum30/2
  "    coeff_q"/1 -> Sum31/1
  Sum34/1 -> Demux10/1
  Sum33/1 -> "   "/1
  Mux29/1 -> "    "/1, "rad-deg     "/1
  Demux10/2 -> Mux29/3
  Demux1/1 -> Mux5/1, "                                                                                                       "/1, Sum3/2
  Transfer Fcn6/1 -> Sum3/1
  Mux5/1 -> Position/1
  Transfer Fcn1/1 -> Sum2/1
  Z_ref/1 -> Transfer Fcn2/1
  Sum3/1 -> Mux37/1
  Demux13/1 -> Sum29/1
  "                                                           "/1 -> Mux29/2
  "             1"/1 -> Demux1/1

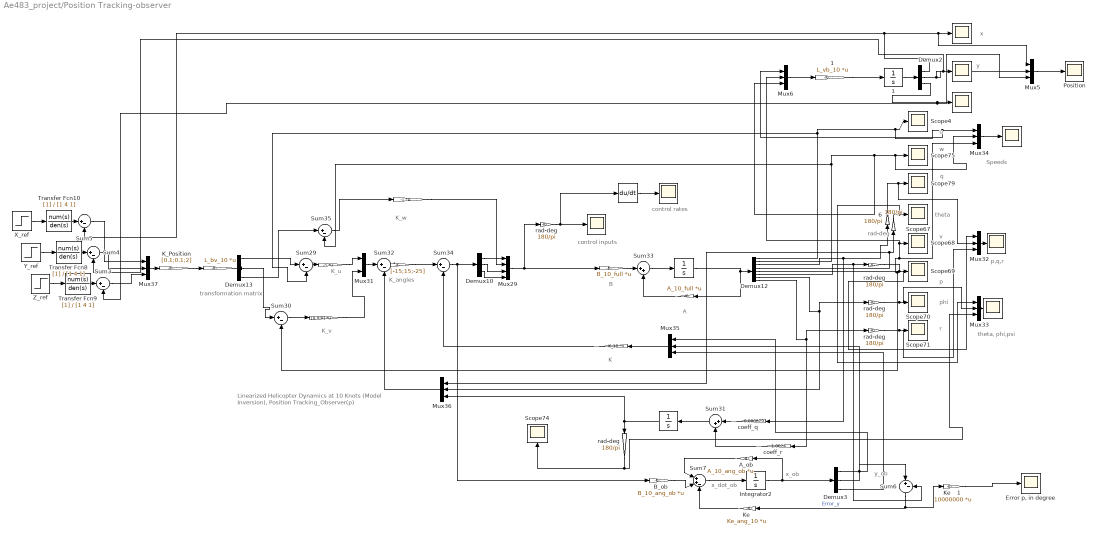
== system Ae483_project/Position Tracking-observer ==
  note: r
  note: theta, phi,psi
  note: rad-deg
  note: phi
  note: Speeds
  note: p,q,r
  note: u
  note: q
  note: v
  note: control rates
  note: K
  note: theta
  note: w
  note: p
  note: B
  note: A
  note: K_w
  note: transformation
      |        matrix
  note: Linearized Helicopter
      | Dynamics at 10 Knots
      | (Model Inversion), Position Tracking_Observer(p)
  note: y
  note: control inputs
  note: K_angles
  note: x
  note: K_u
  note: K_v
  note: x_ob
  note: x_dot_ob
  note: y_ob
  " " : Scope
  "   " : Integrator
  "    " : Gain  Gain=B_10_full  Multiplication=Matrix(K*u)
  "     " : Gain  Gain=180/pi
  "          " : Gain  Gain=A_10_full  Multiplication=Matrix(K*u)
  "                      " : Gain  Gain=K_10  Multiplication=Matrix(K*u)
  "                       " : Gain  Gain=[-15;15;-25]
  "                           " : Gain  Gain=L_bv_10  Multiplication=Matrix(K*u)
  "                                   " : Gain  Gain=-5  Multiplication=Matrix(K*u)
  "                                    " : Gain  Gain=[0.9;0]  Multiplication=Matrix(K*u)
  "                                     " : Derivative
  "                                         " : Scope
  "                                               " : Scope
  "                                                         " : Scope
  "                                                          " : Scope
  "                                                           " : Gain  Gain=-1  Multiplication=Matrix(K*u)
  "                                                             " : Scope
  "                                                                     " : Scope
  "                                                                                           " : Scope
  "                                                                                                           " : Integrator
  "                                                                                                                                                      1" : Gain  Gain=L_vb_10  Multiplication=Matrix(K*u)
  "             1" : Integrator
  "    coeff_q" : Gain  Gain=0.000629
  "    coeff_r" : Gain  Gain=1.0024
  " 6" : Gain  Gain=180/pi
  " rad-deg       " : Gain  Gain=180/pi
  "A_ob   " : Gain  Gain=A_10_ang_ob  Multiplication=Matrix(K*u)
  "B_ob  " : Gain  Gain=B_10_ang_ob  Multiplication=Matrix(K*u)
  Demux{2..3,10,13} (4 alike) : Demux  Outputs=3
  Demux12 : Demux  Outputs=8
  "Error p, in degree" : Scope
  Integrator2 : Integrator
  "K_Position         " : Gain  Gain=[0.1;0.1;2]
  "Ke    " : Gain  Description=K  Gain=Ke_ang_10  Multiplication=Matrix(K*u)
  Ke    1 : Gain  Description=K  Gain=10000000  Multiplication=Matrix(K*u)
  Mux29 : Mux
  Mux31 : Mux  Inputs=2
  Mux{5..6,32..37} (8 alike) : Mux  Inputs=3
  Position : Scope
  Scope{4,67..71,74..75,79} (9 alike) : Scope
  Sum{3..6,29..30,32,34..35} (9 alike) : Sum  Inputs=|+-
  Sum31 : Sum  Inputs=|++
  Sum33 : Sum  Inputs=|++
  Sum7 : Sum  Inputs=|++-
  Transfer Fcn10 : TransferFcn  Denominator=[1 4 1]
  Transfer Fcn8 : TransferFcn  Denominator=[1 4 1]
  Transfer Fcn9 : TransferFcn  Denominator=[1 4 1]
  X_ref : Step  After=50  SampleTime=0
  Y_ref : Step  After=100  SampleTime=0
  Z_ref : Step  After=150  SampleTime=0
  rad-deg : Gain  Gain=180/pi
  "rad-deg  " : Gain  Gain=180/pi
  "rad-deg     " : Gain  Gain=180/pi
  "rad-deg        " : Gain  Gain=180/pi
  wires:
  Demux2/2 -> Mux5/2, Sum4/2, "                                                             "/1
  Demux12/2 -> Mux6/3, Mux34/2, Scope75/1, Sum35/2
  "   "/1 -> Demux12/1, "          "/1
  Demux12/3 -> "    coeff_q"/1, " 6"/1
  "    coeff_r"/1 -> Sum31/2
  Demux10/3 -> Mux29/4
  Integrator2/1 -> Demux3/1, "A_ob   "/1
  Demux12/7 -> rad-deg/1, Mux36/2
  Mux34/1 -> "                                                                     "/1
  Demux13/3 -> Sum35/1
  Demux13/2 -> Sum30/1
  Demux3/1 -> Mux35/1, Sum6/1
  "             1"/1 -> Demux2/1
  Demux2/3 -> Sum3/2, Mux5/3, "                                                          "/1
  Mux35/1 -> "                      "/1
  Sum7/1 -> Integrator2/1
  "    "/1 -> Sum33/1
  Sum6/1 -> "Ke    "/1, Ke    1/1  "Error_y"
  Demux12/8 -> "    coeff_r"/1, " rad-deg       "/1
  Mux33/1 -> "                                               "/1
  " rad-deg       "/1 -> Mux32/3, Scope71/1
  "B_ob  "/1 -> Sum7/2
  Demux12/1 -> Scope4/1, Mux6/1, Mux34/1, Sum29/2
  Sum31/1 -> "                                                                                                           "/1
  "rad-deg  "/1 -> Mux32/1, Scope69/1
  "A_ob   "/1 -> Sum7/1
  Y_ref/1 -> Transfer Fcn8/1
  Demux12/5 -> Mux34/3, Mux6/2, Scope68/1, Sum30/2
  Mux36/1 -> Sum32/2
  "                                                           "/1 -> Mux29/2
  "Ke    "/1 -> Sum7/3
  rad-deg/1 -> Mux33/2, Scope70/1
  Sum29/1 -> "                                   "/1
  "                           "/1 -> Demux13/1
  Mux32/1 -> "                                                         "/1
  "rad-deg     "/1 -> " "/1, "                                     "/1
  Demux3/3 -> Mux35/3
  Sum34/1 -> "B_ob  "/1, Demux10/1
  Mux29/1 -> "    "/1, "rad-deg     "/1
  Mux37/1 -> "K_Position         "/1
  "    coeff_q"/1 -> Sum31/1
  Sum32/1 -> "                       "/1
  Z_ref/1 -> Transfer Fcn9/1
  "K_Position         "/1 -> "                           "/1
  "                                   "/1 -> Mux31/1
  Demux3/2 -> Mux35/2
  "                                    "/1 -> Mux31/2
  Sum3/1 -> Mux37/3
  X_ref/1 -> Transfer Fcn10/1
  Mux6/1 -> "                                                                                                                                                      1"/1
  "                       "/1 -> Sum34/1
  Demux12/6 -> "rad-deg  "/1, Sum6/2
  Transfer Fcn9/1 -> Sum3/1
  Sum30/1 -> "                                    "/1
  Demux10/2 -> Mux29/3
  Demux2/1 -> Mux5/1, "                                                                                           "/1, Sum5/2
  "                                     "/1 -> "                                         "/1
  "          "/1 -> Sum33/2
  Sum33/1 -> "   "/1
  "rad-deg        "/1 -> Scope74/1, Mux33/3
  " 6"/1 -> Mux32/2, Scope79/1
  "                                                                                                                                                      1"/1 -> "             1"/1
  "                                                                                                           "/1 -> "rad-deg        "/1, Mux36/3
  Mux31/1 -> Sum32/1
  "                      "/1 -> Sum34/2
  Demux12/4 -> "     "/1, Mux36/1
  Sum35/1 -> "                                                           "/1
  Transfer Fcn10/1 -> Sum5/1
  Transfer Fcn8/1 -> Sum4/1
  Mux5/1 -> Position/1
  "     "/1 -> Mux33/1, Scope67/1
  Sum5/1 -> Mux37/1
  Demux13/1 -> Sum29/1
  Demux10/1 -> Mux29/1
  Sum4/1 -> Mux37/2
  Ke    1/1 -> "Error p, in degree"/1

== system Ae483_project/Red-With-Controller ==
  note: Reduced Linearized Helicopter
      | Dynamics at 10 Knots
      | With Controller
      | (Model Inversion Method)
  note: Reduced Linearized Helicopter
      | Dynamics at 80 Knots
      | With Controller
      | (Model Inversion Method)
  "         K  " : Gain  Gain=K_80  Multiplication=Matrix(K*u)
  "      Control Deflections    " : Scope
  "     Deg-Rad     " : Gain  Gain=pi/180
  "    K" : Gain  Gain=K_10  Multiplication=Matrix(K*u)
  "   Deg-Rad  " : Gain  Gain=pi/180
  "   r-d    " : Gain  Gain=180/pi
  "  Rad-Deg  " : Gain  Gain=180/pi
  "  Rad-Deg     " : Gain  Gain=180/pi
  "  r-d " : Gain  Gain=180/pi
  " Lat_Cyc" : Step  SampleTime=0
  " Long_Cyc" : Step  SampleTime=0
  " Pedal" : Step  SampleTime=0
  " p,q,r  " : Scope
  " q" : Scope
  " r" : Scope
  "A   " : Gain  Gain=A_80_ang  Multiplication=Matrix(K*u)
  "A     " : Gain  Gain=A_10_ang  Multiplication=Matrix(K*u)
  "B    " : Gain  Gain=B_10_ang  Multiplication=Matrix(K*u)
  "B        " : Gain  Gain=B_80_ang  Multiplication=Matrix(K*u)
  Control Deflections : Scope
  Demux2 : Demux  Outputs=3
  Demux4 : Demux  Outputs=3
  Integrator : Integrator
  "Integrator  " : Integrator
  Lat_Cyc : Step  After=10  SampleTime=0
  Long_Cyc : Step  After=10  SampleTime=0
  Mux{2,4,36..37} (4 alike) : Mux  Inputs=3
  Pedal : Step  After=10  SampleTime=0
  Sum2 : Sum  Inputs=|++
  Sum3 : Sum  Inputs=|+-
  Sum6 : Sum  Inputs=|++
  Sum7 : Sum  Inputs=|+-
  p : Scope
  "p   " : Scope
  p,q,r : Scope
  q : Scope
  r : Scope
  wires:
  "         K  "/1 -> Sum7/2
  Mux2/1 -> "     Deg-Rad     "/1
  Integrator/1 -> "  Rad-Deg  "/1, "    K"/1, "A     "/1
  Mux37/1 -> " p,q,r  "/1
  Pedal/1 -> Mux2/3
  Long_Cyc/1 -> Mux2/1
  Mux4/1 -> "   Deg-Rad  "/1
  " Long_Cyc"/1 -> Mux4/1
  "     Deg-Rad     "/1 -> Sum3/1
  "A     "/1 -> Sum2/2
  "A   "/1 -> Sum6/2
  "B    "/1 -> Sum2/1
  Demux2/2 -> Mux36/2, q/1
  "    K"/1 -> Sum3/2
  " Lat_Cyc"/1 -> Mux4/2
  "   Deg-Rad  "/1 -> Sum7/1
  Demux4/1 -> Mux37/1, "p   "/1
  "B        "/1 -> Sum6/1
  Demux2/3 -> Mux36/3, r/1
  Lat_Cyc/1 -> Mux2/2
  Demux2/1 -> Mux36/1, p/1
  "  Rad-Deg     "/1 -> Demux4/1
  "  Rad-Deg  "/1 -> Demux2/1
  Sum2/1 -> Integrator/1
  Mux36/1 -> p,q,r/1
  Demux4/2 -> Mux37/2, " q"/1
  Sum6/1 -> "Integrator  "/1
  "Integrator  "/1 -> "  Rad-Deg     "/1, "         K  "/1, "A   "/1
  " Pedal"/1 -> Mux4/3
  Demux4/3 -> Mux37/3, " r"/1
  "  r-d "/1 -> Control Deflections/1
  Sum3/1 -> "  r-d "/1, "B    "/1
  "   r-d    "/1 -> "      Control Deflections    "/1
  Sum7/1 -> "   r-d    "/1, "B        "/1

== system Ae483_project/Red-with-LQR ==
  note: Reduced Linearized Helicopter
      | Dynamics at 10 Knots
      | With Controller
      | (LQR Method)
  note: Reduced Linearized Helicopter
      | Dynamics at 80 Knots
      | With Controller
      | (LQR Method)
  "            K  " : Gain  Gain=K_lqr_80  Multiplication=Matrix(K*u)
  "        Deg-Rad      " : Gain  Gain=pi/180
  "       Deg-Rad      " : Gain  Gain=pi/180
  "     K " : Gain  Gain=K_lqr_10  Multiplication=Matrix(K*u)
  "    A   " : Gain  Gain=A_80_ang  Multiplication=Matrix(K*u)
  "    Rad-Deg  " : Gain  Gain=180/pi
  "   B      " : Gain  Gain=B_80_ang  Multiplication=Matrix(K*u)
  "   p,q,r  " : Scope
  "  Control Deflections  " : Scope
  "  Rad-Deg   " : Gain  Gain=180/pi
  "  r  " : Scope
  "  r-d " : Gain  Gain=180/pi
  "  r-d   " : Gain  Gain=180/pi
  " p  " : Scope
  " p,q,r " : Scope
  " q  " : Scope
  "A " : Gain  Gain=A_10_ang  Multiplication=Matrix(K*u)
  "B      " : Gain  Gain=B_10_ang  Multiplication=Matrix(K*u)
  Control Deflections : Scope
  Demux3 : Demux  Outputs=3
  Demux5 : Demux  Outputs=3
  Integrator3 : Integrator
  Integrator5 : Integrator
  "Lat_Cyc " : Step  SampleTime=0
  Lat_Cyc 1 : Step  SampleTime=0
  "Long_Cyc " : Step  SampleTime=0
  Long_Cyc 1 : Step  SampleTime=0
  Mux{3,5,38..39} (4 alike) : Mux  Inputs=3
  "Pedal " : Step  SampleTime=0
  Pedal 1 : Step  SampleTime=0
  Sum4 : Sum  Inputs=|++
  Sum5 : Sum  Inputs=|+-
  Sum8 : Sum  Inputs=|++
  Sum9 : Sum  Inputs=|+-
  "p " : Scope
  "q  " : Scope
  "r  " : Scope
  wires:
  "       Deg-Rad      "/1 -> Sum5/1
  Lat_Cyc 1/1 -> Mux5/2
  "            K  "/1 -> Sum9/2
  Demux3/2 -> Mux38/2, "q  "/1
  Sum5/1 -> "  r-d   "/1, "B      "/1
  "A "/1 -> Sum4/2
  Sum4/1 -> Integrator3/1
  "B      "/1 -> Sum4/1
  Mux3/1 -> "       Deg-Rad      "/1
  "  Rad-Deg   "/1 -> Demux3/1
  "   B      "/1 -> Sum8/1
  "     K "/1 -> Sum5/2
  Demux3/1 -> Mux38/1, "p "/1
  Integrator3/1 -> "  Rad-Deg   "/1, "     K "/1, "A "/1
  Demux5/1 -> Mux39/1, " p  "/1
  Integrator5/1 -> "    Rad-Deg  "/1, "            K  "/1, "    A   "/1
  "        Deg-Rad      "/1 -> Sum9/1
  Sum8/1 -> Integrator5/1
  Demux3/3 -> Mux38/3, "r  "/1
  Demux5/2 -> Mux39/2, " q  "/1
  Mux5/1 -> "        Deg-Rad      "/1
  "Pedal "/1 -> Mux3/3
  "    A   "/1 -> Sum8/2
  Mux38/1 -> " p,q,r "/1
  Pedal 1/1 -> Mux5/3
  "    Rad-Deg  "/1 -> Demux5/1
  Mux39/1 -> "   p,q,r  "/1
  "Long_Cyc "/1 -> Mux3/1
  Long_Cyc 1/1 -> Mux5/1
  "Lat_Cyc "/1 -> Mux3/2
  Demux5/3 -> Mux39/3, "  r  "/1
  "  r-d "/1 -> Control Deflections/1
  Sum9/1 -> "  r-d "/1, "   B      "/1
  "  r-d   "/1 -> "  Control Deflections  "/1
